simulink model "EHB_MOTOR"  (R2023b)
settings: Solver=FixedStepDiscrete  StartTime=0.0  StopTime=inf  FixedStep=0.0001  RelTol=1e-3  EnableMultiTasking=on
undefined symbols (not defined in the file): CAN_EHB_VCU0x125, CAN_EHB_VCU0x126, CAN_id0x120_Data, Cos_Table, Cos_Table1, EHB_DTC_status, R, Sin_BreakPoint, Sin_BreakPoint1, Sin_Table, Sin_Table1, T
libraries: simulink x30
(part 7 of 9)

== system EHB_MOTOR/EHB_MOTOR_PRO/INPUT/AI/EHB_interface/preADC2Presure/vMCU2PIN ==
  note: 运放比例系数
  note: 计算进入主芯片的电压值
  EHB_Presure_AD : Inport
  Constant : Constant  Value=100/101
  Constant1 : Constant  Value=5/4095
  Divide : Product  Inputs=*/
  Multiply : Product
  vPre_MCU2PIN : Outport  VectorParamsAs1DForOutWhenUnconnected=off
  wires:
  Constant/1 -> Divide/2
  Constant1/1 -> Multiply/2
  Multiply/1 -> Divide/1
  Divide/1 -> vPre_MCU2PIN/1
  EHB_Presure_AD/1 -> Multiply/1

== system EHB_MOTOR/EHB_MOTOR_PRO/INPUT/AI/EHB_interface/tempADC2Temp/Filter ==
  In1 : Inport
  Chart : Stateflow chart  TreatAsAtomicUnit=on
  Out1 : Outport  VectorParamsAs1DForOutWhenUnconnected=off
  wires:
  In1/1 -> Chart/1(input)
  Chart/1(output) -> Out1/1

== system EHB_MOTOR/EHB_MOTOR_PRO/INPUT/AI/EHB_interface/tempADC2Temp/Subsystem ==
  EHB_Temp_AD : Inport
  EHB_5vOUT : Inport  Port=2
  Add : Sum  Inputs=+-
  Constant1 : Constant  Value=10
  Divide1 : Product  Inputs=*/
  Multiply : Product
  Saturation : Saturate  UpperLimit=5  LowerLimit=0.1
  Trans_vMCU : Subsystem
  MOS_rTemp : Outport  VectorParamsAs1DForOutWhenUnconnected=off
  wires:
  Multiply/1 -> Divide1/1
  Add/1 -> Saturation/1
  Trans_vMCU/1(TEMP_V) -> Multiply/1, Add/2
  Constant1/1 -> Multiply/2
  EHB_Temp_AD/1 -> Trans_vMCU/1(TEMP_AD)
  Divide1/1 -> MOS_rTemp/1
  Saturation/1 -> Divide1/2
  EHB_5vOUT/1 -> Add/1

== system EHB_MOTOR/EHB_MOTOR_PRO/INPUT/AI/EHB_interface/tempADC2Temp/Subsystem/Trans_vMCU ==
  note: AD通道转换成电压，单位v
  TEMP_AD : Inport
  AD_Trans : Constant  Value=5/4095
  Multiply : Product
  TEMP_V : Outport  VectorParamsAs1DForOutWhenUnconnected=off
  wires:
  TEMP_AD/1 -> Multiply/1
  AD_Trans/1 -> Multiply/2
  Multiply/1 -> TEMP_V/1

== stateflow chart EHB_MOTOR/EHB_MOTOR_PRO/INPUT/AI/EHB_interface/VADC2Cur/Filter/Chart ==
  (default) -> (junction 44)
  (junction 44) -> (junction 41) : {i=0;}
  (junction 41) -> (junction 37) [order 1] : [i<Filter_C]
  (junction 36) -> (junction 41) : {i=i+1;}
  (junction 37) -> (junction 36) : {Filter_Input[i]=Filter_Input[i+1];
      | Filter_Input[Filter_C]=input;
      | sum=sum+Filter_Input[i];
      | output=sum/Filter_C;}
  (junction 41) -> (junction 38) [order 2] : {sum=0;}
  data: input input; output output; i local uint8; Filter_C input uint8; sum local double; Filter_Input local double size=20

== stateflow chart EHB_MOTOR/EHB_MOTOR_PRO/INPUT/AI/EHB_interface/WADC2Cur/Filter/Chart ==
  (default) -> (junction 44)
  (junction 44) -> (junction 41) : {i=0;}
  (junction 41) -> (junction 37) [order 1] : [i<Filter_C]
  (junction 36) -> (junction 41) : {i=i+1;}
  (junction 37) -> (junction 36) : {Filter_Input[i]=Filter_Input[i+1];
      | Filter_Input[Filter_C]=input;
      | sum=sum+Filter_Input[i];
      | output=sum/Filter_C;}
  (junction 41) -> (junction 38) [order 2] : {sum=0;}
  data: input input; output output; i local uint8; Filter_C input uint8; sum local double; Filter_Input local double size=20

== stateflow chart EHB_MOTOR/EHB_MOTOR_PRO/INPUT/AI/EHB_interface/WheelADC2VOLT/Filter/Chart ==
  (default) -> (junction 44)
  (junction 44) -> (junction 41) : {i=0;}
  (junction 41) -> (junction 37) [order 1] : [i<Filter_C]
  (junction 36) -> (junction 41) : {i=i+1;}
  (junction 37) -> (junction 36) : {Filter_Input[i]=Filter_Input[i+1];
      | Filter_Input[Filter_C]=input;
      | sum=sum+Filter_Input[i];
      | output=sum/Filter_C;}
  (junction 41) -> (junction 38) [order 2] : {sum=0;}
  data: input input; output output; i local uint8; Filter_C input uint8; sum local double; Filter_Input local double size=20

== stateflow chart EHB_MOTOR/EHB_MOTOR_PRO/MODE/Chart ==
  state init
    en:EHB_mode=10;
    EHB_35584_en=0;
    EHB_5vOUT_en=0;
    EHB_7189_en=0;
    EHB_CAN_en=0;
    Self_Check_Cmplt=0;
    Pwron_ok=0;
    Zero_Cmplt=0;
    Pwrdwn_ok=0;
    iZero_cnt=0;
    cnt35584=0;
    cnt5vOUT=0;
    AngleZeroCal_cnt=0;
    cnt7189=0;
    cnt5vOUToff=0;
    Fault_pwrdwn_cnt=0;
  state Self_Check
    Self_Check -> (junction 104) [order 1] : {EHB_mode = 1;}
    (junction 104) -> (junction 105) [order 1] : [Self_Check_Sts==1]
    (junction 104) -> (junction 109) [order 2] : {Self_Check_Cmplt = 0;}
    (junction 105) -> (junction 147)
    (junction 147) -> (junction 149) [order 1] : [!ZeroCal_write_ok]
    (junction 147) -> (junction 152) [order 2] : {Self_Check_Cmplt = 1;}
    (junction 149) -> (junction 71)
    (junction 71) -> (junction 75) [order 1] : %电流标零
        | [((Motor_iUzero_AD > 1930)&&(Motor_iUzero_AD < 2070))&&((Motor_iVzero_AD > 1930)&&(Motor_iVzero_AD < 2070))&&((Motor_iWzero_AD > 1930)&&(Motor_iWzero_AD < 2070))]
    (junction 75) -> (junction 79) : {iZero_cnt++;}
    (junction 71) -> (junction 81) [order 2] : {Self_Check_Cmplt = 0;}
    (junction 79) -> (junction 89) [order 1] : [iZero_cnt >= 10]
    (junction 79) -> (junction 94) [order 2]
    (junction 89) -> (junction 91) : {Flash_Ucurrent = Motor_iUzero_AD;
        | Flash_Vcurrent = Motor_iVzero_AD;
        | Flash_Wcurrent = Motor_iWzero_AD;
        | Self_Check_Cmplt = 1;}
    (junction 152) -> (junction 109)
    (junction 81) -> (junction 152)
    (junction 94) -> (junction 81)
    (junction 91) -> (junction 94)
  note: 状态完成标志，复位？
  state Fault
    Fault -> (junction 137) [order 1] : {EHB_mode=6;
        | Fault_pwrdwn_cnt++;}
    (junction 137) -> (junction 139) [order 1] : [Fault_pwrdwn_cnt>=500]
    (junction 137) -> (junction 143) [order 2]
    (junction 139) -> (junction 141) : {EHB_35584_en=0;
        | EHB_5vOUT_en=0;
        | EHB_7189_en=0;
        | EHB_CAN_en=0;
        | Fault_pwrdwn_cnt=0;}
    (junction 141) -> (junction 143)
  state power_on
    power_on -> (junction 7) [order 1] : {EHB_mode=2;
        | EHB_35584_en=1;
        | cnt35584++;}
    (junction 7) -> (junction 10) [order 1] : [cnt35584>=10]
    (junction 7) -> (junction 21) [order 2]
    (junction 10) -> (junction 12) : {EHB_5vOUT_en=1;
        | cnt5vOUT++;}
    (junction 12) -> (junction 14) [order 1] : [cnt5vOUT>=10]
    (junction 12) -> (junction 18) [order 2]
    (junction 14) -> (junction 16) : {EHB_7189_en=1;
        | EHB_CAN_en=1;
        | Pwron_ok=1;}
    (junction 18) -> (junction 21)
    (junction 16) -> (junction 18)
  state power_off
    power_off -> (junction 45) [order 1] : {EHB_mode=4;
        | EHB_7189_en=0;
        | cnt7189++;}
    (junction 45) -> (junction 46) [order 1] : [cnt7189>=10]
    (junction 45) -> (junction 49) [order 2]
    (junction 46) -> (junction 47) : {EHB_5vOUT_en=0;
        | cnt5vOUToff++;}
    (junction 47) -> (junction 48) [order 1] : [cnt5vOUToff>=10]
    (junction 47) -> (junction 50) [order 2]
    (junction 48) -> (junction 51) : {EHB_35584_en=0;
        | cnt7189=0;
        | cnt5vOUToff=0;
        | Pwrdwn_ok=1;}
    (junction 50) -> (junction 49)
    (junction 51) -> (junction 50)
  note: 计数变量，复位？
  state Zero_Cal
    Zero_Cal -> (junction 113) [order 1] : {EHB_mode=3;}
    (junction 113) -> (junction 115) [order 1] : [!ZeroCal_write_ok]
    (junction 113) -> (junction 125) [order 2] : {EHB_AngleZeroCal_Req=0;
        | Zero_Cmplt=1;}
    (junction 115) -> (junction 117) : {AngleZeroCal_cnt++;}
    (junction 117) -> (junction 119) [order 1] : [AngleZeroCal_cnt>=10000]
    (junction 117) -> (junction 123) [order 2] : {EHB_AngleZeroCal_Req=1;
        | Zero_Cmplt=0;}
    (junction 119) -> (junction 121) : {EHB_AngleZeroCal_Req=0;
        | Zero_Cmplt=1;}
    (junction 123) -> (junction 125)
    (junction 121) -> (junction 123)
  state normal
    en:EHB_mode=5;
    EHB_35584_en=1;
    EHB_5vOUT_en=1;
    EHB_7189_en=1;
    EHB_CAN_en=1;
  (default) -> init
  init -> Self_Check : [ignition]
  power_off -> init [order 1] : [Pwrdwn_ok]
  Fault -> init [order 1] : [!ignition]
  Self_Check -> Fault [order 1] : [Fault_Sts]
  Self_Check -> power_on [order 2] : [Self_Check_Cmplt]
  power_on -> Fault [order 2] : [Fault_Sts]
  normal -> Fault [order 1] : [Fault_Sts]
  Zero_Cal -> Fault [order 2] : [Fault_Sts]
  normal -> power_off [order 2] : [!ignition]
  Zero_Cal -> power_off [order 1] : [!ignition]
  power_on -> power_off [order 1] : [!ignition]
  power_on -> Zero_Cal [order 3] : [Pwron_ok]
  Zero_Cal -> normal [order 3] : [Zero_Cmplt]
  data: ignition input boolean; Motor_iUzero_AD input uint16; Motor_iVzero_AD input uint16; Motor_iWzero_AD input uint16; EHB_mode_req input uint8; Self_Check_Sts input uint8; EHB_35584_en output boolean; EHB_5vOUT_en output boolean; EHB_7189_en output boolean; EHB_CAN_en output boolean; EHB_mode output uint8; cnt35584 local uint16; cnt5vOUT local uint16; Fault_Sts input boolean; ZeroCal_write_ok input boolean; Flash_Ucurrent output uint16; Flash_Vcurrent output uint16; Flash_Wcurrent output uint16; iZero_cnt local uint16; Zero_Cmplt local boolean; Pwron_ok local boolean; Pwrdwn_ok local boolean; Self_Check_Cmplt local boolean; AngleZeroCal_cnt local uint16; EHB_AngleZeroCal_Req output uint8; cnt7189 local uint16; cnt5vOUToff local uint16; Fault_pwrdwn_cnt local uint16

== stateflow chart EHB_MOTOR/EHB_MOTOR_PRO/DIAG/AngleSensorDiag/Subsystem/ErrorSignalCount ==
  state errClear
    en:AngleSensorSignalOverride=0;
    Counter=0;
  state errConfirm
    en:AngleSensorSignalOverride=0;
    du:Counter++;
  state errTrue
    en:AngleSensorSignalOverride=1;
    Counter=0;
  (default) -> errClear
  errClear -> errConfirm : [AngleSensorSignal==1]
  errConfirm -> errClear [order 2] : [AngleSensorSignal==0]
  errTrue -> errClear : [Recover==1]
  errConfirm -> errTrue [order 1] : [Counter >= AngleSensorSignalOverride_C]
  data: AngleSensorSignal input boolean; AngleSensorSignalOverride output boolean; AngleSensorSignalOverride_C input uint16; Counter local uint16; Recover input uint8

== stateflow chart EHB_MOTOR/EHB_MOTOR_PRO/DIAG/AngleSensorDiag/Subsystem1/ErrorSignalCount ==
  state errClear
    en:AngleSensorSignalLost=0;
    Counter=0;
  state errConfirm
    en:AngleSensorSignalLost=0;
    du:Counter++;
  state errTrue
    en:AngleSensorSignalLost=1;
    Counter=0;
  (default) -> errClear
  errClear -> errConfirm : [AngleSensorSignal==1]
  errConfirm -> errClear [order 2] : [AngleSensorSignal==0]
  errTrue -> errClear : [Recover==1]
  errConfirm -> errTrue [order 1] : [Counter >= AngleSensorSignalLost_C]
  data: AngleSensorSignal input boolean; AngleSensorSignalLost output boolean; AngleSensorSignalLost_C input uint16; Counter local uint16; Recover input uint8

== stateflow chart EHB_MOTOR/EHB_MOTOR_PRO/DIAG/AngleSensorDiag/Subsystem2/ErrorSignalCount ==
  state errClear
    en:AngleSensorNoCal=0;
    Counter=0;
  state errConfirm
    en:AngleSensorNoCal=0;
    du:Counter++;
  state errTrue
    en:AngleSensorNoCal=1;
    Counter=0;
  (default) -> errClear
  errClear -> errConfirm : [AngleSensorSignal==1]
  errConfirm -> errClear [order 2] : [AngleSensorSignal==0]
  errTrue -> errClear : [Recover==1]
  errConfirm -> errTrue [order 1] : [Counter >= AngleSensorNoCal_C]
  data: AngleSensorSignal input boolean; AngleSensorNoCal output boolean; AngleSensorNoCal_C input uint16; Counter local uint16; Recover input uint8

== stateflow chart EHB_MOTOR/EHB_MOTOR_PRO/DIAG/MotorDiag/Subsystem/ErrorSignalCount ==
  state errClear
    en:MotorCircuitCurrentOverride=0;
    Counter=0;
  state errConfirm
    en:MotorCircuitCurrentOverride=0;
    du:Counter++;
  state errTrue
    en:MotorCircuitCurrentOverride=1;
    Counter=0;
  (default) -> errClear
  errClear -> errConfirm : [MotorCircuitCurrent==1]
  errConfirm -> errClear [order 2] : [MotorCircuitCurrent==0]
  errTrue -> errClear : [Recover==1]
  errConfirm -> errTrue [order 1] : [Counter >= MotorCircuitCurrentOverride_C]
  data: MotorCircuitCurrent input boolean; MotorCircuitCurrentOverride output boolean; MotorCircuitCurrentOverride_C input uint8; Counter local uint8; Recover input uint8

== stateflow chart EHB_MOTOR/EHB_MOTOR_PRO/DIAG/PressureSensorDiag/Subsystem/ErrorSignalCount ==
  state errClear
    en:PressureSensorSignalOverride=0;
    Counter=0;
  state errConfirm
    en:PressureSensorSignalOverride=0;
    du:Counter++;
  state errTrue
    en:PressureSensorSignalOverride=1;
    Counter=0;
  (default) -> errClear
  errClear -> errConfirm : [PressureSensorSignal==1]
  errConfirm -> errClear [order 1] : [PressureSensorSignal==0]
  errTrue -> errClear : [Recover==1]
  errConfirm -> errTrue [order 2] : [Counter >= PressureSensorSignalOverride_C]
  data: PressureSensorSignal input boolean; PressureSensorSignalOverride output boolean; PressureSensorSignalOverride_C input uint16; Counter local uint16; Recover input uint8

== stateflow chart EHB_MOTOR/EHB_MOTOR_PRO/DIAG/PressureSensorDiag/Subsystem1/ErrorSignalCount ==
  state errClear
    en:PressureSensorSignalLost=0;
    Counter=0;
  state errConfirm
    en:PressureSensorSignalLost=0;
    du:Counter++;
  state errTrue
    en:PressureSensorSignalLost=1;
    Counter=0;
  (default) -> errClear
  errClear -> errConfirm : [PressureSensorSignal==1]
  errConfirm -> errClear [order 1] : [PressureSensorSignal==0]
  errTrue -> errClear : [Recover==1]
  errConfirm -> errTrue [order 2] : [Counter >= PressureSensorSignalLost_C]
  data: PressureSensorSignal input boolean; PressureSensorSignalLost output boolean; PressureSensorSignalLost_C input uint16; Counter local uint16; Recover input uint8

== stateflow chart EHB_MOTOR/EHB_MOTOR_PRO/DIAG/PressureSensorDiag/Subsystem2/ErrorSignalCount ==
  state errClear
    en:PressureSensorNoCal=0;
    Counter=0;
  state errConfirm
    en:PressureSensorNoCal=0;
    du:Counter++;
  state errTrue
    en:PressureSensorNoCal=1;
    Counter=0;
  (default) -> errClear
  errClear -> errConfirm : [PressureSensorSignal==1]
  errConfirm -> errClear [order 1] : [PressureSensorSignal==0]
  errTrue -> errClear : [Recover==1]
  errConfirm -> errTrue [order 2] : [Counter >= PressureSensorNoCal_C]
  data: PressureSensorSignal input boolean; PressureSensorNoCal output boolean; PressureSensorNoCal_C input uint16; Counter local uint16; Recover input uint8

== stateflow chart EHB_MOTOR/EHB_MOTOR_PRO/OUTPUT/CAN_pack/Msg_0x125 ==
  (default) -> (junction 8)
  (junction 8) -> (junction 10) : {EHB_BrakingResponse_0x125[0]=(EHBStatus&0x01)|((BrakeCondition&0x03)<<1)|((EHBFaultLevel&0x0F)<<3);
      | EHB_BrakingResponse_0x125[1]=ActualPressure;
      | EHB_BrakingResponse_0x125[2]=0x00;
      | EHB_BrakingResponse_0x125[3]=0x00;
      | EHB_BrakingResponse_0x125[4]=0x00;
      | EHB_BrakingResponse_0x125[5]=0x00;
      | EHB_BrakingResponse_0x125[6]=(RollingCounter&0x0F)<<4;
      | EHB_BrakingResponse_0x125[7]=(EHB_BrakingResponse_0x125[0])^(EHB_BrakingResponse_0x125[1])^(EHB_BrakingResponse_0x125[2])^(EHB_BrakingResponse_0x125[3])^...
      |                                                         (EHB_BrakingResponse_0x125[4])^(EHB_BrakingResponse_0x125[5])^(EHB_BrakingResponse_0x125[6]);}
  data: EHB_BrakingResponse_0x125 output uint8 size=8; EHBStatus input uint8; ActualPressure input uint8; BrakeCondition input uint8; EHBFaultLevel input uint8; RollingCounter input uint8

== stateflow chart EHB_MOTOR/EHB_MOTOR_PRO/INPUT/AI/EHB_interface/preADC2Presure/Filter/Chart ==
  (default) -> (junction 44)
  (junction 44) -> (junction 41) : {i=0;}
  (junction 41) -> (junction 37) [order 1] : [i<Filter_C]
  (junction 36) -> (junction 41) : {i=i+1;}
  (junction 37) -> (junction 36) : {Filter_Input[i]=Filter_Input[i+1];
      | Filter_Input[Filter_C]=input;
      | sum=sum+Filter_Input[i];
      | output=sum/Filter_C;}
  (junction 41) -> (junction 38) [order 2] : {sum=0;}
  data: input input; output output; i local uint8; Filter_C input uint8; sum local double; Filter_Input local double size=20

== stateflow chart EHB_MOTOR/EHB_MOTOR_PRO/OUTPUT/CAN_pack/RollingCounter ==
  state Counter1
    du: counter++;
  state Counter2
    en: counter = 0;
    ex: counter = 1;
  (default) -> Counter1
  Counter1 -> Counter2 : [counter == 15]
  Counter2 -> Counter1 : [counter < 15]
  data: counter output uint8

== stateflow chart EHB_MOTOR/EHB_MOTOR_PRO/INPUT/AI/EHB_interface/tempADC2Temp/Filter/Chart ==
  (default) -> (junction 44)
  (junction 44) -> (junction 41) : {i=0;}
  (junction 41) -> (junction 37) [order 1] : [i<Filter_C]
  (junction 36) -> (junction 41) : {i=i+1;}
  (junction 37) -> (junction 36) : {Filter_Input[i]=Filter_Input[i+1];
      | Filter_Input[Filter_C]=input;
      | sum=sum+Filter_Input[i];
      | output=sum/Filter_C;}
  (junction 41) -> (junction 38) [order 2] : {sum=0;}
  data: input input; output output; i local uint8; Filter_C input uint8; sum local double; Filter_Input local double size=20

== stateflow chart EHB_MOTOR/EPB_CTRL/Subsystem1/EPB_interface/12vADC2VOLT/Filter/Chart ==
  (default) -> (junction 44)
  (junction 44) -> (junction 41) : {i=0;}
  (junction 41) -> (junction 37) [order 1] : [i<Filter_C]
  (junction 36) -> (junction 41) : {i=i+1;}
  (junction 37) -> (junction 36) : {Filter_Input[i]=Filter_Input[i+1];
      | Filter_Input[Filter_C]=input;
      | sum=sum+Filter_Input[i];
      | output=sum/Filter_C;}
  (junction 41) -> (junction 38) [order 2] : {sum=0;}
  data: input input; output output; i local uint8; Filter_C input uint8; sum local double; Filter_Input local double size=20

== stateflow chart EHB_MOTOR/EPB_CTRL/Subsystem1/EPB_interface/EPB1DC2Cur/Filter/Chart ==
  (default) -> (junction 44)
  (junction 44) -> (junction 41) : {i=0;}
  (junction 41) -> (junction 37) [order 1] : [i<Filter_C]
  (junction 36) -> (junction 41) : {i=i+1;}
  (junction 37) -> (junction 36) : {Filter_Input[i]=Filter_Input[i+1];
      | Filter_Input[Filter_C]=input;
      | sum=sum+Filter_Input[i];
      | output=sum/Filter_C;}
  (junction 41) -> (junction 38) [order 2] : {sum=0;}
  data: input input; output output; i local uint8; Filter_C input uint8; sum local double; Filter_Input local double size=20

== stateflow chart EHB_MOTOR/EHB_MOTOR_PRO/OUTPUT/CAN_pack/Chart ==
  (default) -> (junction 24)
  (junction 24) -> (junction 26) : {EHB_Diagnostics_0x126[0] = BrkReqWarn|(PFolwFltLv1<<1)|(PCtrlVibLv1<<2)|(NTCFltLv1<<3)|(NTCFltLv2<<4)|(PSnsrFlt<<5)|(OverTempWarn<<6)|(USplyLowLv1<<7);
      | EHB_Diagnostics_0x126[1] = USplyHighLv1|(PFolwFltLv2<<1)|(PCtrlVibLv2<<2)|(LoadMismatchFlt<<3)|(CANBusOff<<4)|(OverIFlt<<5)|(ISnsrFlt<<6)|(USplyLowLv2<<7);
      | EHB_Diagnostics_0x126[2] = USplyHighLv2|(PwrSwtFlt<<1)|(PwrDrvrFlt<<2)|(MotPosnFlt<<3);
      | EHB_Diagnostics_0x126[3] = 0x00;
      | EHB_Diagnostics_0x126[4] = 0x00;
      | EHB_Diagnostics_0x126[5] = 0x00;
      | EHB_Diagnostics_0x126[6] = EHB_SoftwareVersion;
      | EHB_Diagnostics_0x126[7] = EHB_HardwareVersion;}
  data: EHB_Diagnostics_0x126 output uint8 size=8; BrkReqWarn input uint8; PFolwFltLv1 input uint8; PCtrlVibLv1 input uint8; NTCFltLv1 input uint8; NTCFltLv2 input uint8; PSnsrFlt input uint8; OverTempWarn input uint8; USplyLowLv1 input uint8; USplyHighLv1 input uint8; PFolwFltLv2 input uint8; PCtrlVibLv2 input uint8; LoadMismatchFlt input uint8; CANBusOff input uint8; OverIFlt input uint8; ISnsrFlt input uint8; USplyLowLv2 input uint8; USplyHighLv2 input uint8; PwrSwtFlt input uint8; PwrDrvrFlt input uint8; MotPosnFlt input uint8; EHB_SoftwareVersion input uint8; EHB_HardwareVersion input uint8

== stateflow chart EHB_MOTOR/EPB_CTRL/Subsystem1/EPB_interface/EPB2DC2Cur/Filter/Chart ==
  (default) -> (junction 44)
  (junction 44) -> (junction 41) : {i=0;}
  (junction 41) -> (junction 37) [order 1] : [i<Filter_C]
  (junction 36) -> (junction 41) : {i=i+1;}
  (junction 37) -> (junction 36) : {Filter_Input[i]=Filter_Input[i+1];
      | Filter_Input[Filter_C]=input;
      | sum=sum+Filter_Input[i];
      | output=sum/Filter_C;}
  (junction 41) -> (junction 38) [order 2] : {sum=0;}
  data: input input; output output; i local uint8; Filter_C input uint8; sum local double; Filter_Input local double size=20

== stateflow chart EHB_MOTOR/EPB_CTRL/Subsystem1/EPB_interface/EPB_7181PreDriver1/Filter/Chart ==
  (default) -> (junction 44)
  (junction 44) -> (junction 41) : {i=0;}
  (junction 41) -> (junction 37) [order 1] : [i<Filter_C]
  (junction 36) -> (junction 41) : {i=i+1;}
  (junction 37) -> (junction 36) : {Filter_Input[i]=Filter_Input[i+1];
      | Filter_Input[Filter_C]=input;
      | sum=sum+Filter_Input[i];
      | output=sum/Filter_C;}
  (junction 41) -> (junction 38) [order 2] : {sum=0;}
  data: input input; output output; i local uint8; Filter_C input uint8; sum local double; Filter_Input local double size=20

== stateflow chart EHB_MOTOR/EPB_CTRL/Subsystem1/EPB_interface/EPB_7181PreDriver2/Filter/Chart ==
  (default) -> (junction 44)
  (junction 44) -> (junction 41) : {i=0;}
  (junction 41) -> (junction 37) [order 1] : [i<Filter_C]
  (junction 36) -> (junction 41) : {i=i+1;}
  (junction 37) -> (junction 36) : {Filter_Input[i]=Filter_Input[i+1];
      | Filter_Input[Filter_C]=input;
      | sum=sum+Filter_Input[i];
      | output=sum/Filter_C;}
  (junction 41) -> (junction 38) [order 2] : {sum=0;}
  data: input input; output output; i local uint8; Filter_C input uint8; sum local double; Filter_Input local double size=20

== stateflow chart EHB_MOTOR/EPB_CTRL/Subsystem1/EPB_interface/EPB_APBSwitch1/Filter/Chart ==
  (default) -> (junction 44)
  (junction 44) -> (junction 41) : {i=0;}
  (junction 41) -> (junction 37) [order 1] : [i<Filter_C]
  (junction 36) -> (junction 41) : {i=i+1;}
  (junction 37) -> (junction 36) : {Filter_Input[i]=Filter_Input[i+1];
      | Filter_Input[Filter_C]=input;
      | sum=sum+Filter_Input[i];
      | output=sum/Filter_C;}
  (junction 41) -> (junction 38) [order 2] : {sum=0;}
  data: input input; output output; i local uint8; Filter_C input uint8; sum local double; Filter_Input local double size=20

== stateflow chart EHB_MOTOR/EPB_CTRL/Subsystem1/EPB_interface/EPB_APBSwitch2/Filter/Chart ==
  (default) -> (junction 44)
  (junction 44) -> (junction 41) : {i=0;}
  (junction 41) -> (junction 37) [order 1] : [i<Filter_C]
  (junction 36) -> (junction 41) : {i=i+1;}
  (junction 37) -> (junction 36) : {Filter_Input[i]=Filter_Input[i+1];
      | Filter_Input[Filter_C]=input;
      | sum=sum+Filter_Input[i];
      | output=sum/Filter_C;}
  (junction 41) -> (junction 38) [order 2] : {sum=0;}
  data: input input; output output; i local uint8; Filter_C input uint8; sum local double; Filter_Input local double size=20

== stateflow chart EHB_MOTOR/EPB_CTRL/Subsystem1/EPB_interface/EPB_APBSwitch3/Filter/Chart ==
  (default) -> (junction 44)
  (junction 44) -> (junction 41) : {i=0;}
  (junction 41) -> (junction 37) [order 1] : [i<Filter_C]
  (junction 36) -> (junction 41) : {i=i+1;}
  (junction 37) -> (junction 36) : {Filter_Input[i]=Filter_Input[i+1];
      | Filter_Input[Filter_C]=input;
      | sum=sum+Filter_Input[i];
      | output=sum/Filter_C;}
  (junction 41) -> (junction 38) [order 2] : {sum=0;}
  data: input input; output output; i local uint8; Filter_C input uint8; sum local double; Filter_Input local double size=20

== stateflow chart EHB_MOTOR/EPB_CTRL/Subsystem1/EPB_interface/EPB_APBSwitch4/Filter/Chart ==
  (default) -> (junction 44)
  (junction 44) -> (junction 41) : {i=0;}
  (junction 41) -> (junction 37) [order 1] : [i<Filter_C]
  (junction 36) -> (junction 41) : {i=i+1;}
  (junction 37) -> (junction 36) : {Filter_Input[i]=Filter_Input[i+1];
      | Filter_Input[Filter_C]=input;
      | sum=sum+Filter_Input[i];
      | output=sum/Filter_C;}
  (junction 41) -> (junction 38) [order 2] : {sum=0;}
  data: input input; output output; i local uint8; Filter_C input uint8; sum local double; Filter_Input local double size=20

== stateflow chart EHB_MOTOR/EPB_CTRL/Subsystem1/EPB_interface/tempADC2Temp/Filter/Chart ==
  (default) -> (junction 44)
  (junction 44) -> (junction 41) : {i=0;}
  (junction 41) -> (junction 37) [order 1] : [i<Filter_C]
  (junction 36) -> (junction 41) : {i=i+1;}
  (junction 37) -> (junction 36) : {Filter_Input[i]=Filter_Input[i+1];
      | Filter_Input[Filter_C]=input;
      | sum=sum+Filter_Input[i];
      | output=sum/Filter_C;}
  (junction 41) -> (junction 38) [order 2] : {sum=0;}
  data: input input; output output; i local uint8; Filter_C input uint8; sum local double; Filter_Input local double size=20

== stateflow chart EHB_MOTOR/EPB_CTRL/Subsystem1/EPB_interface/tempADC2Temp1/Filter/Chart ==
  (default) -> (junction 44)
  (junction 44) -> (junction 41) : {i=0;}
  (junction 41) -> (junction 37) [order 1] : [i<Filter_C]
  (junction 36) -> (junction 41) : {i=i+1;}
  (junction 37) -> (junction 36) : {Filter_Input[i]=Filter_Input[i+1];
      | Filter_Input[Filter_C]=input;
      | sum=sum+Filter_Input[i];
      | output=sum/Filter_C;}
  (junction 41) -> (junction 38) [order 2] : {sum=0;}
  data: input input; output output; i local uint8; Filter_C input uint8; sum local double; Filter_Input local double size=20

== stateflow chart EHB_MOTOR/EHB_MOTOR_PRO/INPUT/CAN/0x120 ==
  (default) -> (junction 1)
  (junction 1) -> (junction 3) : {BrakingEnable=CAN_id0x120_Data[0]&0x0F;
      | ParkingBrakeActive=CAN_id0x120_Data[0]&0xF0;
      | Brake_AimPressure=0.1*(CAN_id0x120_Data[1]);
      | RollingCounter=CAN_id0x120_Data[6]&0xF0;
      | Checksum=CAN_id0x120_Data[7];}
  data: CAN_id0x120_Data input uint8 size=8; BrakingEnable output uint8; ParkingBrakeActive output uint8; Brake_AimPressure output single; RollingCounter output uint8; Checksum output uint8

== stateflow chart EHB_MOTOR/EHB_MOTOR_PRO/DIAG/MotorDiag/Subsystem1/ErrorSignalCount ==
  state errClear
    en:MotorTempOverride=0;
    Counter=0;
  state errConfirm
    en:MotorTempOverride=0;
    du:Counter++;
  state errTrue
    en:MotorTempOverride=1;
    Counter=0;
  (default) -> errClear
  errClear -> errConfirm : [MotorTemp==1]
  errConfirm -> errClear [order 2] : [MotorTemp==0]
  errTrue -> errClear : [Recover==1]
  errConfirm -> errTrue [order 1] : [Counter >= MotorTempOverride_C]
  data: MotorTemp input boolean; MotorTempOverride output boolean; MotorTempOverride_C input uint8; Counter local uint8; Recover input uint8

== stateflow chart EHB_MOTOR/EHB_MOTOR_PRO/DIAG/MotorDiag/Subsystem2/ErrorSignalCount ==
  state errClear
    en:MotorCurrentOverride=0;
    Counter=0;
  state errConfirm
    en:MotorCurrentOverride=0;
    du:Counter++;
  state errTrue
    en:MotorCurrentOverride=1;
    Counter=0;
  (default) -> errClear
  errClear -> errConfirm : [MotorCurrent==1]
  errConfirm -> errClear [order 2] : [MotorCurrent==0]
  errTrue -> errClear : [Recover==1]
  errConfirm -> errTrue [order 1] : [Counter >= MotorCurrentOverride_C]
  data: MotorCurrent input boolean; MotorCurrentOverride output boolean; MotorCurrentOverride_C input uint8; Counter local uint8; Recover input uint8

== stateflow chart EHB_MOTOR/EHB_MOTOR_PRO/DIAG/EHBDiag/Subsystem/ErrorSignalCount ==
  state errClear
    en:EHBVoltageMAX=0;
    Counter=0;
  state errConfirm
    en:EHBVoltageMAX=0;
    du:Counter++;
  state errTrue
    en:EHBVoltageMAX=1;
    Counter=0;
  (default) -> errClear
  errClear -> errConfirm : [EHBVoltage==1]
  errConfirm -> errClear [order 2] : [EHBVoltage==0]
  errTrue -> errClear : [Recover==1]
  errConfirm -> errTrue [order 1] : [Counter >= EHBVoltageMAX_C]
  data: EHBVoltage input boolean; EHBVoltageMAX output boolean; EHBVoltageMAX_C input uint16; Counter local uint16; Recover input uint8

== stateflow chart EHB_MOTOR/EHB_MOTOR_PRO/DIAG/EHBDiag/Subsystem/ErrorSignalCount1 ==
  state errClear
    en:EHBVoltageMIN=0;
    Counter=0;
  state errConfirm
    en:EHBVoltageMIN=0;
    du:Counter++;
  state errTrue
    en:EHBVoltageMIN=1;
    Counter=0;
  (default) -> errClear
  errClear -> errConfirm : [EHBVoltage==1]
  errConfirm -> errClear [order 2] : [EHBVoltage==0]
  errTrue -> errClear : [Recover==1]
  errConfirm -> errTrue [order 1] : [Counter >= EHBVoltageMIN_C]
  data: EHBVoltage input boolean; EHBVoltageMIN output boolean; EHBVoltageMIN_C input uint16; Counter local uint16; Recover input uint8

== stateflow chart EHB_MOTOR/EPB_CTRL/EPB_Diag/EPB_vBATDiag/Subsystem/ErrorSignalCount ==
  state errClear
    en:EPBVoltageMAX=0;
    Counter=0;
  state errConfirm
    en:EPBVoltageMAX=0;
    du:Counter++;
  state errTrue
    en:EPBVoltageMAX=1;
    Counter=0;
  (default) -> errClear
  errClear -> errConfirm : [EPBVoltage==1]
  errConfirm -> errClear [order 2] : [EPBVoltage==0]
  errTrue -> errClear : [Recover==1]
  errConfirm -> errTrue [order 1] : [Counter >= EPBVoltageMAX_C]
  data: EPBVoltage input boolean; EPBVoltageMAX output boolean; EPBVoltageMAX_C input uint16; Counter local uint8; Recover input uint8

== stateflow chart EHB_MOTOR/EPB_CTRL/EPB_Diag/EPB_vBATDiag/Subsystem/ErrorSignalCount1 ==
  state errClear
    en:EPBVoltageMIN=0;
    Counter=0;
  state errConfirm
    en:EPBVoltageMIN=0;
    du:Counter++;
  state errTrue
    en:EPBVoltageMIN=1;
    Counter=0;
  (default) -> errClear
  errClear -> errConfirm : [EPBVoltage==1]
  errConfirm -> errClear [order 2] : [EPBVoltage==0]
  errTrue -> errClear : [Recover==1]
  errConfirm -> errTrue [order 1] : [Counter >= EPBVoltageMIN_C]
  data: EPBVoltage input boolean; EPBVoltageMIN output boolean; EPBVoltageMIN_C input uint16; Counter local uint8; Recover input uint8

== stateflow chart EHB_MOTOR/EHB_MOTOR_PRO/DIAG/LogicVoltageDiag/Subsystem/ErrorSignalCount ==
  state errClear
    en:LogicVoltageMAX=0;
    Counter=0;
  state errConfirm
    en:LogicVoltageMAX=0;
    du:Counter++;
  state errTrue
    en:LogicVoltageMAX=1;
    Counter=0;
  (default) -> errClear
  errClear -> errConfirm : [LogicVoltage==1]
  errConfirm -> errClear [order 2] : [LogicVoltage==0]
  errTrue -> errClear : [Recover==1]
  errConfirm -> errTrue [order 1] : [Counter >= LogicVoltageMAX_C]
  data: LogicVoltage input boolean; LogicVoltageMAX output boolean; LogicVoltageMAX_C input uint16; Counter local uint16; Recover input uint8

== stateflow chart EHB_MOTOR/EHB_MOTOR_PRO/DIAG/LogicVoltageDiag/Subsystem/ErrorSignalCount1 ==
  state errClear
    en:LogicVoltageMIN=0;
    Counter=0;
  state errConfirm
    en:LogicVoltageMIN=0;
    du:Counter++;
  state errTrue
    en:LogicVoltageMIN=1;
    Counter=0;
  (default) -> errClear
  errClear -> errConfirm : [LogicVoltage==1]
  errConfirm -> errClear [order 2] : [LogicVoltage==0]
  errTrue -> errClear : [Recover==1]
  errConfirm -> errTrue [order 1] : [Counter >= LogicVoltageMIN_C]
  data: LogicVoltage input boolean; LogicVoltageMIN output boolean; LogicVoltageMIN_C input uint16; Counter local uint16; Recover input uint8

== stateflow chart EHB_MOTOR/EHB_MOTOR_PRO/DIAG/KL15VoltageDiag/Subsystem/ErrorSignalCount ==
  state errClear
    en:KL15VoltageMAX=0;
    Counter=0;
  state errConfirm
    en:KL15VoltageMAX=0;
    du:Counter++;
  state errTrue
    en:KL15VoltageMAX=1;
    Counter=0;
  state errRestore
    en:KL15VoltageMAX=1;
    du:Counter++;
  (default) -> errClear
  errClear -> errConfirm : [KL15Voltage==1]
  errConfirm -> errClear [order 2] : [KL15Voltage==0]
  errRestore -> errClear : [Counter >= KL15VoltageMAX_C]
  errTrue -> errClear [order 1] : [Recover==1]
  errConfirm -> errTrue [order 1] : [Counter >= KL15VoltageMAX_C]
  errTrue -> errRestore [order 2] : [KL15Voltage==0]
  data: KL15Voltage input boolean; KL15VoltageMAX output boolean; KL15VoltageMAX_C input uint16; Counter local uint16; Recover input uint8

== stateflow chart EHB_MOTOR/EHB_MOTOR_PRO/DIAG/KL15VoltageDiag/Subsystem/ErrorSignalCount1 ==
  state errClear
    en:KL15VoltageMIN=0;
    Counter=0;
  state errConfirm
    en:KL15VoltageMIN=0;
    du:Counter++;
  state errTrue
    en:KL15VoltageMIN=1;
    Counter=0;
  state errRestore
    en:KL15VoltageMIN=1;
    du:Counter++;
  (default) -> errClear
  errClear -> errConfirm : [KL15Voltage==1]
  errConfirm -> errClear [order 2] : [KL15Voltage==0]
  errRestore -> errClear : [Counter >= KL15VoltageMIN_C]
  errTrue -> errClear [order 1] : [Recover==1]
  errConfirm -> errTrue [order 1] : [Counter >= KL15VoltageMIN_C]
  errTrue -> errRestore [order 2] : [KL15Voltage==0]
  data: KL15Voltage input boolean; KL15VoltageMIN output boolean; KL15VoltageMIN_C input uint16; Counter local uint16; Recover input uint8

== stateflow chart EHB_MOTOR/EHB_MOTOR_PRO/DIAG/CurrentSensorDiag/Subsystem/ErrorSignalCount ==
  state errClear
    en:CurrentSensorUOverride=0;
    Counter=0;
  state errConfirm
    en:CurrentSensorUOverride=0;
    du:Counter++;
  state errTrue
    en:CurrentSensorUOverride=1;
    Counter=0;
  (default) -> errClear
  errClear -> errConfirm : [CurrentSensorU==1]
  errConfirm -> errClear [order 1] : [CurrentSensorU==0]
  errTrue -> errClear : [Recover==1]
  errConfirm -> errTrue [order 2] : [Counter >= CurrentSensorUOverride_C]
  data: CurrentSensorU input boolean; CurrentSensorUOverride output boolean; CurrentSensorUOverride_C input uint16; Counter local uint16; Recover input uint8

== stateflow chart EHB_MOTOR/EHB_MOTOR_PRO/DIAG/CurrentSensorDiag/Subsystem1/ErrorSignalCount ==
  state errClear
    en:CurrentSensorVOverride=0;
    Counter=0;
  state errConfirm
    en:CurrentSensorVOverride=0;
    du:Counter++;
  state errTrue
    en:CurrentSensorVOverride=1;
    Counter=0;
  (default) -> errClear
  errClear -> errConfirm : [CurrentSensorV==1]
  errConfirm -> errClear [order 1] : [CurrentSensorV==0]
  errTrue -> errClear : [Recover==1]
  errConfirm -> errTrue [order 2] : [Counter >= CurrentSensorVOverride_C]
  data: CurrentSensorV input boolean; CurrentSensorVOverride output boolean; CurrentSensorVOverride_C input uint16; Counter local uint16; Recover input uint8

== stateflow chart EHB_MOTOR/EHB_MOTOR_PRO/DIAG/CurrentSensorDiag/Subsystem2/ErrorSignalCount ==
  state errClear
    en:CurrentSensorWOverride=0;
    Counter=0;
  state errConfirm
    en:CurrentSensorWOverride=0;
    du:Counter++;
  state errTrue
    en:CurrentSensorWOverride=1;
    Counter=0;
  (default) -> errClear
  errClear -> errConfirm : [CurrentSensorW==1]
  errConfirm -> errClear [order 1] : [CurrentSensorW==0]
  errTrue -> errClear : [Recover==1]
  errConfirm -> errTrue [order 2] : [Counter >= CurrentSensorWOverride_C]
  data: CurrentSensorW input boolean; CurrentSensorWOverride output boolean; CurrentSensorWOverride_C input uint16; Counter local uint16; Recover input uint8

== stateflow chart EHB_MOTOR/EHB_MOTOR_PRO/DIAG/TempDiag/Subsystem1/ErrorSignalCount ==
  state errClear
    en:TempSensorOverride=0;
    Counter=0;
  state errConfirm
    en:TempSensorOverride=0;
    du:Counter++;
  state errTrue
    en:TempSensorOverride=1;
    Counter=0;
  (default) -> errClear
  errClear -> errConfirm : [TempSensor==1]
  errConfirm -> errClear [order 1] : [TempSensor==0]
  errTrue -> errClear : [Recover==1]
  errConfirm -> errTrue [order 2] : [Counter >= TempSensorOverride_C]
  data: TempSensor input boolean; TempSensorOverride output boolean; TempSensorOverride_C input uint16; Counter local uint16; Recover input uint8

== stateflow chart EHB_MOTOR/EHB_MOTOR_PRO/DIAG/5vDiag/Chart ==
  (default) -> (junction 3) : {cnt++;}
  (junction 3) -> (junction 5) [order 1] : [cnt>=10]
  (junction 3) -> (junction 9) [order 2]
  (junction 5) -> (junction 7) : {cnt=0;
      | task_20ms;}
  (junction 7) -> (junction 9)
  data: cnt local uint16
  events: task_20ms output FUNCTION_CALL_EVENT

== stateflow chart EHB_MOTOR/EHB_MOTOR_PRO/DIAG/5vDiag/Subsystem/ErrorSignalCount1 ==
  state errClear
    en:V5VoltageMIN=0;
    Counter=0;
  state errConfirm
    en:V5VoltageMIN=0;
    du:Counter++;
  state errTrue
    en:V5VoltageMIN=1;
    Counter=0;
  (default) -> errClear
  errClear -> errConfirm : [V5Voltage==1]
  errConfirm -> errClear [order 2] : [V5Voltage==0]
  errTrue -> errClear : [Recover==1]
  errConfirm -> errTrue [order 1] : [Counter >= V5VoltageMIN_C]
  data: V5Voltage input boolean; V5VoltageMIN output boolean; V5VoltageMIN_C input uint16; Counter local uint16; Recover input uint8

== stateflow chart EHB_MOTOR/EHB_MOTOR_PRO/DIAG/AngleSensorDiag/Chart ==
  (default) -> (junction 3) : {cnt++;}
  (junction 3) -> (junction 5) [order 1] : [cnt>=100]
  (junction 3) -> (junction 9) [order 2]
  (junction 5) -> (junction 7) : {cnt=0;
      | task_200ms;}
  (junction 7) -> (junction 9)
  data: cnt local uint16
  events: task_200ms output FUNCTION_CALL_EVENT

== stateflow chart EHB_MOTOR/EHB_MOTOR_PRO/DIAG/AngleSensorDiag/Chart1 ==
  (default) -> (junction 3) : {cnt++;}
  (junction 3) -> (junction 5) [order 1] : [cnt>=100]
  (junction 3) -> (junction 9) [order 2]
  (junction 5) -> (junction 7) : {cnt=0;
      | task_200ms;}
  (junction 7) -> (junction 9)
  data: cnt local uint16
  events: task_200ms output FUNCTION_CALL_EVENT

== stateflow chart EHB_MOTOR/EHB_MOTOR_PRO/DIAG/Chip7189Diag/Subsystem/ErrorSignalCount ==
  state errClear
    en:Chip7189Err=0;
    Counter=0;
  state errConfirm
    en:Chip7189Err=0;
    du:Counter++;
  state errTrue
    en:Chip7189Err=1;
    Counter=0;
  (default) -> errClear
  errClear -> errConfirm : [Chip7189==1]
  errConfirm -> errClear [order 2] : [Chip7189==0]
  errTrue -> errClear : [Recover==1]
  errConfirm -> errTrue [order 1] : [Counter >= Chip7189Err_C]
  data: Chip7189 input boolean; Chip7189Err output boolean; Chip7189Err_C input uint16; Counter local uint16; Recover input uint8

== stateflow chart EHB_MOTOR/EHB_MOTOR_PRO/DIAG/AngleSensorDiag/Chart2 ==
  (default) -> (junction 3) : {cnt++;}
  (junction 3) -> (junction 5) [order 1] : [cnt>=100]
  (junction 3) -> (junction 9) [order 2]
  (junction 5) -> (junction 7) : {cnt=0;
      | task_200ms;}
  (junction 7) -> (junction 9)
  data: cnt local uint16
  events: task_200ms output FUNCTION_CALL_EVENT

== stateflow chart EHB_MOTOR/EHB_MOTOR_PRO/DIAG/PressureSensorDiag/Chart ==
  (default) -> (junction 3) : {cnt++;}
  (junction 3) -> (junction 5) [order 1] : [cnt>=100]
  (junction 3) -> (junction 9) [order 2]
  (junction 5) -> (junction 7) : {cnt=0;
      | task_200ms;}
  (junction 7) -> (junction 9)
  data: cnt local uint16
  events: task_200ms output FUNCTION_CALL_EVENT

== stateflow chart EHB_MOTOR/EHB_MOTOR_PRO/DIAG/PressureSensorDiag/Chart1 ==
  (default) -> (junction 3) : {cnt++;}
  (junction 3) -> (junction 5) [order 1] : [cnt>=100]
  (junction 3) -> (junction 9) [order 2]
  (junction 5) -> (junction 7) : {cnt=0;
      | task_200ms;}
  (junction 7) -> (junction 9)
  data: cnt local uint16
  events: task_200ms output FUNCTION_CALL_EVENT

== stateflow chart EHB_MOTOR/EHB_MOTOR_PRO/DIAG/PressureSensorDiag/Chart2 ==
  (default) -> (junction 3) : {cnt++;}
  (junction 3) -> (junction 5) [order 1] : [cnt>=100]
  (junction 3) -> (junction 9) [order 2]
  (junction 5) -> (junction 7) : {cnt=0;
      | task_200ms;}
  (junction 7) -> (junction 9)
  data: cnt local uint16
  events: task_200ms output FUNCTION_CALL_EVENT

== stateflow chart EHB_MOTOR/EPB_CTRL/EPB_Diag/EPBOverheatDiag/Subsystem1/ErrorSignalCount ==
  state errConfirm
    en:EPBTempOverride=0;
    du:Counter++;
  state errClear
    en:EPBTempOverride=0;
    Counter=0;
  state errTrue
    en:EPBTempOverride=1;
    Counter=0;
  (default) -> errClear
  errClear -> errConfirm : [EPBTemp==1]
  errConfirm -> errClear [order 2] : [EPBTemp==0]
  errTrue -> errClear : [Recover==1]
  errConfirm -> errTrue [order 1] : [Counter >= EPBTempOverride_C]
  data: EPBTemp input boolean; EPBTempOverride output boolean; EPBTempOverride_C input uint16; Counter local uint8; Recover input uint8

== stateflow chart EHB_MOTOR/EHB_MOTOR_PRO/DIAG/SpeedSensorDiag/Subsystem/ErrorSignalCount ==
  state errClear
    en:SpeedSensorOverride=0;
    Counter=0;
  state errConfirm
    en:SpeedSensorOverride=0;
    du:Counter++;
  state errTrue
    en:SpeedSensorOverride=1;
    Counter=0;
  (default) -> errClear
  errClear -> errConfirm : [SpeedSensor==1]
  errConfirm -> errClear [order 2] : [SpeedSensor==0]
  errTrue -> errClear : [Recover==1]
  errConfirm -> errTrue [order 1] : [Counter >= SpeedSensorOverride_C]
  data: SpeedSensor input boolean; SpeedSensorOverride output boolean; SpeedSensorOverride_C input uint16; Counter local uint16; Recover input uint8

== stateflow chart EHB_MOTOR/EPB_CTRL/EPB_Diag/EPBCurrentDiag/Subsystem/ErrorSignalCount ==
  state errClear
    en:EPBCurrentOverride=0;
    Counter=0;
  state errConfirm
    en:EPBCurrentOverride=0;
    du:Counter++;
  state errTrue
    en:EPBCurrentOverride=1;
    Counter=0;
  (default) -> errClear
  errClear -> errConfirm : [EPBCurrent==1]
  errConfirm -> errClear [order 2] : [EPBCurrent==0]
  errTrue -> errClear : [Recover==1]
  errConfirm -> errTrue [order 1] : [Counter >= EPBCurrentOverride_C]
  data: EPBCurrent input boolean; EPBCurrentOverride output boolean; EPBCurrentOverride_C input uint16; Counter local uint8; Recover input uint8

== stateflow chart EHB_MOTOR/EHB_MOTOR_PRO/DIAG/PressureSensorDiag/Subsystem/ErrorSignalCount1 ==
  state errClear
    en:PressureSensorSignalOverride=0;
    Counter=0;
  state errConfirm
    en:PressureSensorSignalOverride=0;
    du:Counter++;
  state errTrue
    en:PressureSensorSignalOverride=1;
    Counter=0;
  (default) -> errClear
  errClear -> errConfirm : [PressureSensorSignal==1]
  errConfirm -> errClear [order 1] : [PressureSensorSignal==0]
  errTrue -> errClear : [Recover==1]
  errConfirm -> errTrue [order 2] : [Counter >= PressureSensorSignalOverride_C]
  data: PressureSensorSignal input boolean; PressureSensorSignalOverride output boolean; PressureSensorSignalOverride_C input uint16; Counter local uint16; Recover input uint8

== stateflow chart EHB_MOTOR/EHB_MOTOR_PRO/DIAG/EHBDiag/Subsystem/ErrorSignalCount2 ==
  state errClear
    en:EHBVoltageMIN=0;
    Counter=0;
  state errConfirm
    en:EHBVoltageMIN=0;
    du:Counter++;
  state errTrue
    en:EHBVoltageMIN=1;
    Counter=0;
  (default) -> errClear
  errClear -> errConfirm : [EHBVoltage==1]
  errConfirm -> errClear [order 2] : [EHBVoltage==0]
  errTrue -> errClear : [Recover==1]
  errConfirm -> errTrue [order 1] : [Counter >= EHBVoltageMIN_C]
  data: EHBVoltage input boolean; EHBVoltageMIN output boolean; EHBVoltageMIN_C input uint16; Counter local uint16; Recover input uint8

== stateflow chart EHB_MOTOR/EHB_MOTOR_PRO/DIAG/EHBDiag/Subsystem/ErrorSignalCount3 ==
  state errClear
    en:EHBVoltageMAX=0;
    Counter=0;
  state errConfirm
    en:EHBVoltageMAX=0;
    du:Counter++;
  state errTrue
    en:EHBVoltageMAX=1;
    Counter=0;
  (default) -> errClear
  errClear -> errConfirm : [EHBVoltage==1]
  errConfirm -> errClear [order 2] : [EHBVoltage==0]
  errTrue -> errClear : [Recover==1]
  errConfirm -> errTrue [order 1] : [Counter >= EHBVoltageMAX_C]
  data: EHBVoltage input boolean; EHBVoltageMAX output boolean; EHBVoltageMAX_C input uint16; Counter local uint16; Recover input uint8

== stateflow chart EHB_MOTOR/EHB_MOTOR_PRO/DIAG/MotorDiag/Chart ==
  (default) -> (junction 3) : {cnt++;}
  (junction 3) -> (junction 5) [order 1] : [cnt>=100]
  (junction 3) -> (junction 9) [order 2]
  (junction 5) -> (junction 7) : {cnt=0;
      | task_200ms;}
  (junction 7) -> (junction 9)
  data: cnt local uint16
  events: task_200ms output FUNCTION_CALL_EVENT

== stateflow chart EHB_MOTOR/EHB_MOTOR_PRO/DIAG/MotorDiag/Chart1 ==
  (default) -> (junction 3) : {cnt++;}
  (junction 3) -> (junction 5) [order 1] : [cnt>=100]
  (junction 3) -> (junction 9) [order 2]
  (junction 5) -> (junction 7) : {cnt=0;
      | task_200ms;}
  (junction 7) -> (junction 9)
  data: cnt local uint16
  events: task_200ms output FUNCTION_CALL_EVENT

== stateflow chart EHB_MOTOR/EHB_MOTOR_PRO/DIAG/MotorDiag/Chart2 ==
  (default) -> (junction 3) : {cnt++;}
  (junction 3) -> (junction 5) [order 1] : [cnt>=100]
  (junction 3) -> (junction 9) [order 2]
  (junction 5) -> (junction 7) : {cnt=0;
      | task_200ms;}
  (junction 7) -> (junction 9)
  data: cnt local uint16
  events: task_200ms output FUNCTION_CALL_EVENT

== stateflow chart EHB_MOTOR/EHB_MOTOR_PRO/DIAG/EHBDiag/Chart ==
  (default) -> (junction 3) : {cnt++;}
  (junction 3) -> (junction 5) [order 1] : [cnt>=100]
  (junction 3) -> (junction 9) [order 2]
  (junction 5) -> (junction 7) : {cnt=0;
      | task_200ms;}
  (junction 7) -> (junction 9)
  data: cnt local uint16
  events: task_200ms output FUNCTION_CALL_EVENT

== stateflow chart EHB_MOTOR/EPB_CTRL/EPB_Diag/EPB_vBATDiag/Chart ==
  (default) -> (junction 3) : {cnt++;}
  (junction 3) -> (junction 5) [order 1] : [cnt>=100]
  (junction 3) -> (junction 9) [order 2]
  (junction 5) -> (junction 7) : {cnt=0;
      | task_200ms;}
  (junction 7) -> (junction 9)
  data: cnt local uint16
  events: task_200ms output FUNCTION_CALL_EVENT

== stateflow chart EHB_MOTOR/EHB_MOTOR_PRO/DIAG/LogicVoltageDiag/Chart ==
  (default) -> (junction 3) : {cnt++;}
  (junction 3) -> (junction 5) [order 1] : [cnt>=100]
  (junction 3) -> (junction 9) [order 2]
  (junction 5) -> (junction 7) : {cnt=0;
      | task_200ms;}
  (junction 7) -> (junction 9)
  data: cnt local uint16
  events: task_200ms output FUNCTION_CALL_EVENT

== stateflow chart EHB_MOTOR/EHB_MOTOR_PRO/DIAG/KL15VoltageDiag/Chart ==
  (default) -> (junction 3) : {cnt++;}
  (junction 3) -> (junction 5) [order 1] : [cnt>=100]
  (junction 3) -> (junction 9) [order 2]
  (junction 5) -> (junction 7) : {cnt=0;
      | task_200ms;}
  (junction 7) -> (junction 9)
  data: cnt local uint16
  events: task_200ms output FUNCTION_CALL_EVENT

== stateflow chart EHB_MOTOR/EHB_MOTOR_PRO/DIAG/CurrentSensorDiag/Chart ==
  (default) -> (junction 3) : {cnt++;}
  (junction 3) -> (junction 5) [order 1] : [cnt>=100]
  (junction 3) -> (junction 9) [order 2]
  (junction 5) -> (junction 7) : {cnt=0;
      | task_200ms;}
  (junction 7) -> (junction 9)
  data: cnt local uint16
  events: task_200ms output FUNCTION_CALL_EVENT

== stateflow chart EHB_MOTOR/EHB_MOTOR_PRO/DIAG/CurrentSensorDiag/Chart1 ==
  (default) -> (junction 3) : {cnt++;}
  (junction 3) -> (junction 5) [order 1] : [cnt>=100]
  (junction 3) -> (junction 9) [order 2]
  (junction 5) -> (junction 7) : {cnt=0;
      | task_200ms;}
  (junction 7) -> (junction 9)
  data: cnt local uint16
  events: task_200ms output FUNCTION_CALL_EVENT

== stateflow chart EHB_MOTOR/EHB_MOTOR_PRO/DIAG/CurrentSensorDiag/Chart2 ==
  (default) -> (junction 3) : {cnt++;}
  (junction 3) -> (junction 5) [order 1] : [cnt>=100]
  (junction 3) -> (junction 9) [order 2]
  (junction 5) -> (junction 7) : {cnt=0;
      | task_200ms;}
  (junction 7) -> (junction 9)
  data: cnt local uint16
  events: task_200ms output FUNCTION_CALL_EVENT

== stateflow chart EHB_MOTOR/EHB_MOTOR_PRO/DIAG/TempDiag/Chart ==
  (default) -> (junction 3) : {cnt++;}
  (junction 3) -> (junction 5) [order 1] : [cnt>=100]
  (junction 3) -> (junction 9) [order 2]
  (junction 5) -> (junction 7) : {cnt=0;
      | task_200ms;}
  (junction 7) -> (junction 9)
  data: cnt local uint16
  events: task_200ms output FUNCTION_CALL_EVENT

== stateflow chart EHB_MOTOR/EHB_MOTOR_PRO/DIAG/Chip7189Diag/Chart ==
  (default) -> (junction 3) : {cnt++;}
  (junction 3) -> (junction 5) [order 1] : [cnt>=10]
  (junction 3) -> (junction 9) [order 2]
  (junction 5) -> (junction 7) : {cnt=0;
      | task_20ms;}
  (junction 7) -> (junction 9)
  data: cnt local uint16
  events: task_20ms output FUNCTION_CALL_EVENT

== stateflow chart EHB_MOTOR/EPB_CTRL/EPB_Diag/EPBOverheatDiag/Chart ==
  (default) -> (junction 3) : {cnt++;}
  (junction 3) -> (junction 5) [order 1] : [cnt>=100]
  (junction 3) -> (junction 9) [order 2]
  (junction 5) -> (junction 7) : {cnt=0;
      | task_200ms;}
  (junction 7) -> (junction 9)
  data: cnt local uint16
  events: task_200ms output FUNCTION_CALL_EVENT

== stateflow chart EHB_MOTOR/EHB_MOTOR_PRO/DIAG/SpeedSensorDiag/Chart ==
  (default) -> (junction 3) : {cnt++;}
  (junction 3) -> (junction 5) [order 1] : [cnt>=100]
  (junction 3) -> (junction 9) [order 2]
  (junction 5) -> (junction 7) : {cnt=0;
      | task_200ms;}
  (junction 7) -> (junction 9)
  data: cnt local uint16
  events: task_200ms output FUNCTION_CALL_EVENT

== stateflow chart EHB_MOTOR/EPB_CTRL/EPB_Diag/EPBCurrentDiag/Chart ==
  (default) -> (junction 3) : {cnt++;}
  (junction 3) -> (junction 5) [order 1] : [cnt>=100]
  (junction 3) -> (junction 9) [order 2]
  (junction 5) -> (junction 7) : {cnt=0;
      | task_200ms;}
  (junction 7) -> (junction 9)
  data: cnt local uint16
  events: task_200ms output FUNCTION_CALL_EVENT

== stateflow chart EHB_MOTOR/EHB_MOTOR_PRO/OUTPUT/FUALT_HANDLE/Chart ==
  (default) -> (junction 5)
  (junction 5) -> (junction 7) [order 1] : [Pressure_CMD != 0]
  (junction 5) -> (junction 11) [order 2] : {keep_Pre_cnt = 0;}
  (junction 7) -> (junction 9) : {keep_Pre_cnt++;}
  (junction 9) -> (junction 11) [order 2]
  (junction 9) -> (junction 13) [order 1] : [PreREQ_Changed_flag]
  (junction 11) -> (junction 18)
  (junction 13) -> (junction 15) : {keep_Pre_cnt = 0;}
  (junction 18) -> (junction 21) [order 1] : [keep_Pre_cnt > 5000]
  (junction 15) -> (junction 18)
  (junction 21) -> (junction 23) : {Pressure_Req = 3;}
  (junction 18) -> (junction 25) [order 2] : {Pressure_Req = Pressure_CMD;}
  (junction 23) -> (junction 25)
  data: keep_Pre_cnt local uint16; Pressure_CMD input; PreREQ_Changed_flag input; Pressure_Req output single

== stateflow chart EHB_MOTOR/EPB_CTRL/EPB_CTRL/Chart ==
  state INIT
    en:EPB_PWMout=0;
    EPB_dir_state=0;
    EPB_clamp_cnt=0;
    EPB_release_cnt=0;
  state RELEASE
    RELEASE -> (junction 28) [order 1] : {EPB_PWMout=5250;
        | EPB_dir_state=2;
        | EPB_release_cnt++;}
    (junction 28) -> (junction 29) [order 1] : [EPB_release_cnt>=EPB_tiRelease_C]
    (junction 28) -> (junction 30) [order 2]
    (junction 29) -> (junction 31) : {EPB_PWMout=0;
        | EPB_dir_state=0;
        | EPB_release_cnt=0;
        | Release_ok=1;
        | Clamp_ok=0;}
    (junction 31) -> (junction 30)
  state CLAMP
    CLAMP -> (junction 12) [order 1] : {EPB_PWMout=5250;
        | EPB_dir_state=1;
        | EPB_clamp_cnt++;}
    (junction 12) -> (junction 14) [order 1] : [(EPB_clamp_cnt>=EPB_tiClamp_C)&&(EPB1_iAct>=EPB1_iAct_C)&&(EPB2_iAct>=EPB2_iAct_C)]
    (junction 12) -> (junction 21) [order 2]
    (junction 14) -> (junction 16) : {EPB_PWMout=0;
        | EPB_dir_state=0;
        | EPB_clamp_cnt=0;
        | Clamp_ok=1;
        | Release_ok=0;}
    (junction 16) -> (junction 21)
  state CLAMP_Cmplt
    en:EPB_PWMout=0;
    EPB_dir_state=0;
    EPB_clamp_cnt=0;
  (default) -> INIT
  RELEASE -> INIT [order 1] : [Release_ok]
  INIT -> CLAMP [order 1] : [EPB_Ctrl_Req==1]
  INIT -> RELEASE [order 2] : [EPB_Ctrl_Req==2]
  CLAMP_Cmplt -> RELEASE : [EPB_Ctrl_Req==2]
  CLAMP -> CLAMP_Cmplt [order 1] : [Clamp_ok]
  data: EPB_Ctrl_Req input uint8; EPB1_iAct input; EPB2_iAct input; EPB_clamp_cnt local uint16; EPB_release_cnt local uint16; EPB_PWMout output uint16; EPB_dir_state output uint8; EPB_tiClamp_C input uint16; EPB_tiRelease_C input uint16; EPB1_iAct_C input single; EPB2_iAct_C input single; Clamp_ok output boolean; Release_ok output boolean
